simulink model "Process"  (R2022b)
settings: Solver=VariableStepAuto  StartTime=0.0  StopTime=5000  RelTol=1e-3
model workspace (MAT data in the model file):
  A = Simulink.Parameter
  A.DataType = 'auto'
  A.Complexity = 'real'
  A.Dimensions = [0 0]
  Q = Simulink.Parameter
  Q.DataType = 'auto'
  Q.Complexity = 'real'
  Q.Dimensions = [0 0]
values from neighbouring files (symbols this model uses):
  A = (pi)*D^2    (= 314.159265359)    [Equations.m]
  Q = l/sec    (= 1000)    [Equations.m]
undefined symbols (not defined in the file or in its folder): i, m
libraries: dspnetwork x4
settings Model: Creator=karnbongkotboonriong  LastModifiedBy=mluser

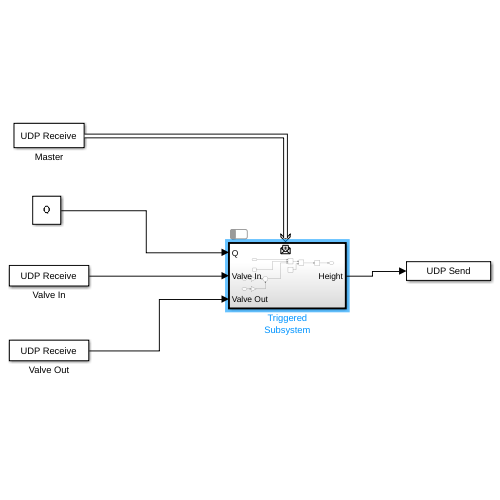
[thumbnail: Simulink's stored preview of the top-level diagram]
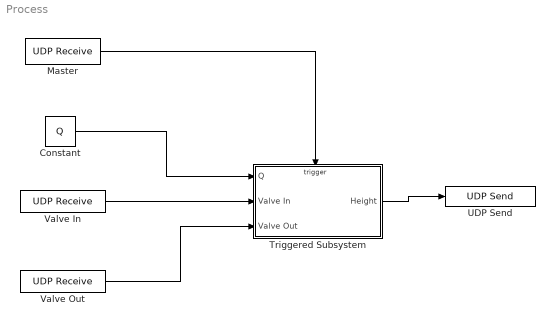
== system Process ==
  Constant : Constant  Value=Q
  Master : dspnetwork/UDP Receive  localURL='0.0.0.0'  localPort=25000  remoteURL='0.0.0.0'  remotePort=-1  recvBufferSize=8192  dims=255  signalDatatype=uint8  isComplex=off  isVarSize=on  showBlockingTime=off  blockingTime=0  sampletime=1  blockPlatform=[]
      settings: LibrarySourceBlock=dspsrcs4/UDP Receive
  Triggered Subsystem : Subsystem  InputPortMessageModes=i,i,i,m  TreatAsAtomicUnit=on  ScheduleAs=Aperiodic partition  PartitionName=TEMP_PRECOMP_PARTITION_NAME_MessageTriggeredSubsystem
  UDP Send : dspnetwork/UDP Send  remoteURL='127.0.0.1'  remotePort=25000  localURL='0.0.0.0'  localPortSource=Automatically determine  localPort=-1  sendBufferSize=8192  sampletime=-1  blockPlatform=[]  separateLengthPort=0
      settings: LibrarySourceBlock=dspsnks4/UDP Send
  Valve In : dspnetwork/UDP Receive  localURL='0.0.0.0'  localPort=25000  remoteURL='0.0.0.0'  remotePort=-1  recvBufferSize=8192  dims=255  signalDatatype=uint8  isComplex=off  isVarSize=on  showBlockingTime=off  blockingTime=0  sampletime=1  blockPlatform=[]
      settings: LibrarySourceBlock=dspsrcs4/UDP Receive
  Valve Out : dspnetwork/UDP Receive  localURL='0.0.0.0'  localPort=25000  remoteURL='0.0.0.0'  remotePort=-1  recvBufferSize=8192  dims=255  signalDatatype=uint8  isComplex=off  isVarSize=on  showBlockingTime=off  blockingTime=0  sampletime=1  blockPlatform=[]
      settings: LibrarySourceBlock=dspsrcs4/UDP Receive
  wires:
  Triggered Subsystem/1(Height) -> UDP Send/1
  Master/1 -> Triggered Subsystem/Trigger
  Constant/1 -> Triggered Subsystem/1(Q)
  Valve In/1 -> Triggered Subsystem/2(Valve In)
  Valve Out/1 -> Triggered Subsystem/3(Valve Out)

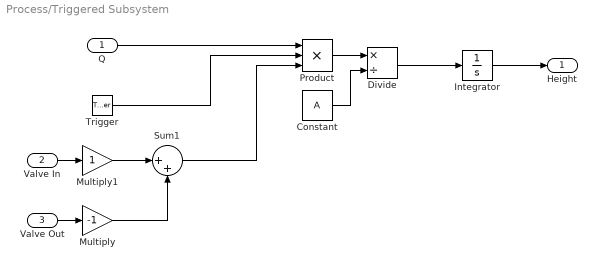
== system Process/Triggered Subsystem ==
  Q : Inport
  Valve In : Inport  Port=2
  Valve Out : Inport  Port=3
  Trigger : TriggerPort  TriggerType=message  VariantControl=(inherit)
  Constant : Constant  Value=A
  Divide : Product  Inputs=*/
  Integrator : Integrator
  Multiply : Gain  Gain=-1
  Multiply1 : Gain
  Product : Product  Inputs=3
  Sum1 : Sum  Inputs=|++
  Height : Outport
  wires:
  Divide/1 -> Integrator/1
  Product/1 -> Divide/1
  Constant/1 -> Divide/2
  Q/1 -> Product/1
  Integrator/1 -> Height/1
  Trigger/1 -> Product/2
  Sum1/1 -> Product/3
  Valve In/1 -> Multiply1/1
  Valve Out/1 -> Multiply/1
  Multiply1/1 -> Sum1/1
  Multiply/1 -> Sum1/2
